simulink model "observer"  (R2014b)
settings: Solver=ode45  StartTime=0.0  StopTime=10.0  RelTol=1e-3
values from neighbouring files (symbols this model uses):
  A11 = A2(1,1)    [zad_8.m]
  A12 = A2(1,2:3)    [zad_8.m]
  A21 = A2(2:3,1)    [zad_8.m]
  A22 = A2(2:3,2:3)    [zad_8.m]
  B_1 = B2(1,1)    [zad_8.m]
  B_2 = B2(2:3,1)    [zad_8.m]
  L = acker(A22',A12', [z2 z3])'    [zad_8.m]
  x0_observer = [ 0 0 ]    [zad_8.m]
undefined symbols (not defined in the file or in its folder): A2, B2, K, Tp, x0
settings Model: Creator=Konrad  LastModifiedBy=Konrad

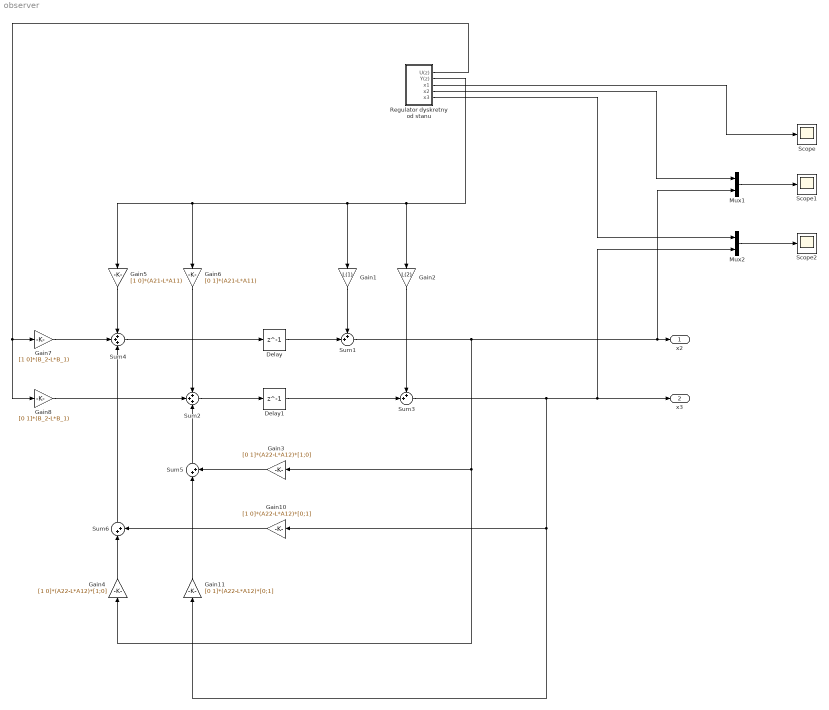
== system observer ==
  Delay : Delay  DelayLength=1  InitialCondition=x0_observer(1)  SampleTime=Tp
  Delay1 : Delay  DelayLength=1  InitialCondition=x0_observer(2)  SampleTime=Tp
  Gain1 : Gain  Gain=L(1)
  Gain10 : Gain  Gain=[1 0]*(A22-L*A12)*[0;1]
  Gain11 : Gain  Gain=[0 1]*(A22-L*A12)*[0;1]
  Gain2 : Gain  Gain=L(2)
  Gain3 : Gain  Gain=[0 1]*(A22-L*A12)*[1;0]
  Gain4 : Gain  Gain=[1 0]*(A22-L*A12)*[1;0]
  Gain5 : Gain  Gain=[1 0]*(A21-L*A11)
  Gain6 : Gain  Gain=[0 1]*(A21-L*A11)
  Gain7 : Gain  Gain=[1 0]*(B_2-L*B_1)
  Gain8 : Gain  Gain=[0 1]*(B_2-L*B_1)
  Mux1 : Mux  Inputs=2
  Mux2 : Mux  Inputs=2
  Regulator dyskretny od stanu : Subsystem
  Scope : Scope
  Scope1 : Scope
  Scope2 : Scope
      settings: SaveName=ScopeData2
  Sum1 : Sum  Inputs=++|
  Sum2 : Sum  Inputs=+++
  Sum3 : Sum  Inputs=++|
  Sum4 : Sum  Inputs=+++
  Sum5 : Sum  Inputs=|++
  Sum6 : Sum  Inputs=|++
  x2 : Outport
  x3 : Outport  Port=2
  wires:
  Delay1/1 -> Sum3/2
  Delay/1 -> Sum1/2
  Regulator dyskretny od stanu/2(Y(z)) -> Gain5/1, Gain6/1, Gain1/1, Gain2/1
  Regulator dyskretny od stanu/1(U(z)) -> Gain8/1, Gain7/1
  Gain3/1 -> Sum5/2
  Gain10/1 -> Sum6/2
  Sum3/1 -> Gain11/1, Gain10/1, Mux2/2, x3/1
  Sum1/1 -> Gain4/1, Gain3/1, Mux1/2, x2/1
  Gain4/1 -> Sum6/1
  Gain11/1 -> Sum5/1
  Gain1/1 -> Sum1/1
  Gain2/1 -> Sum3/1
  Gain5/1 -> Sum4/1
  Gain7/1 -> Sum4/2
  Sum4/1 -> Delay/1
  Sum6/1 -> Sum4/3
  Gain6/1 -> Sum2/1
  Sum2/1 -> Delay1/1
  Sum5/1 -> Sum2/3
  Gain8/1 -> Sum2/2
  Mux1/1 -> Scope1/1
  Mux2/1 -> Scope2/1
  Regulator dyskretny od stanu/4(x2) -> Mux1/1
  Regulator dyskretny od stanu/5(x3) -> Mux2/1
  Regulator dyskretny od stanu/3(x1) -> Scope/1

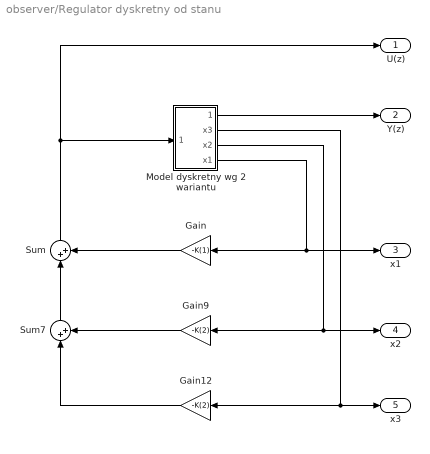
== system observer/Regulator dyskretny od stanu ==
  Gain : Gain  Gain=-K(1)
  Gain12 : Gain  Gain=-K(2)
  Gain9 : Gain  Gain=-K(2)
  Model dyskretny wg 2 wariantu : Subsystem
  Sum : Sum  Inputs=|++
  Sum7 : Sum  Inputs=|++
  U(z) : Outport
  Y(z) : Outport  Port=2
  x1 : Outport  Port=3
  x2 : Outport  Port=4
  x3 : Outport  Port=5
  wires:
  Model dyskretny wg 2 wariantu/1(Y(z)) -> Y(z)/1
  Sum/1 -> U(z)/1, Model dyskretny wg 2 wariantu/1(U(z))
  Gain9/1 -> Sum7/2
  Model dyskretny wg 2 wariantu/4(x1) -> x1/1, Gain/1
  Model dyskretny wg 2 wariantu/2(x3) -> Gain12/1, x3/1
  Sum7/1 -> Sum/1
  Model dyskretny wg 2 wariantu/3(x2) -> Gain9/1, x2/1
  Gain12/1 -> Sum7/1
  Gain/1 -> Sum/2

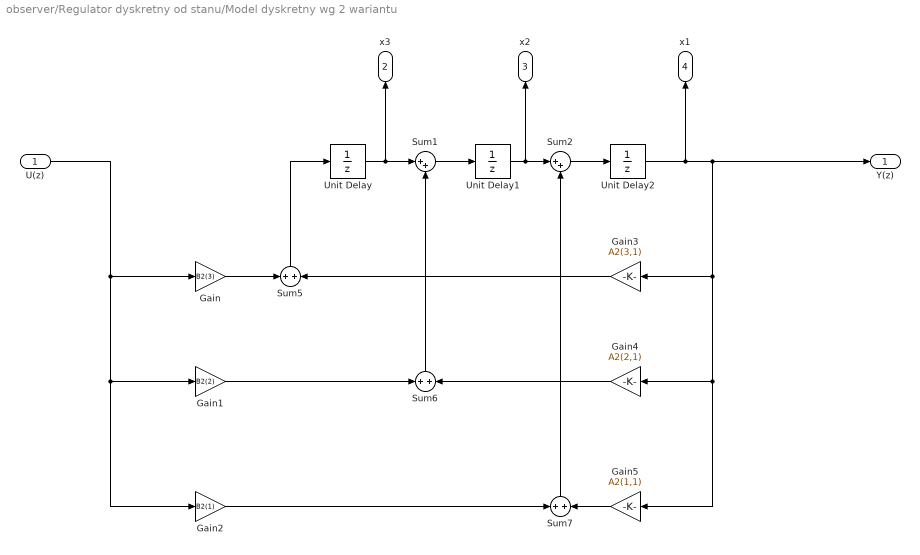
== system observer/Regulator dyskretny od stanu/Model dyskretny wg 2 wariantu ==
  U(z) : Inport
  Gain : Gain  Gain=B2(3)
  Gain1 : Gain  Gain=B2(2)
  Gain2 : Gain  Gain=B2(1)
  Gain3 : Gain  Gain=A2(3,1)
  Gain4 : Gain  Gain=A2(2,1)
  Gain5 : Gain  Gain=A2(1,1)
  Sum1 : Sum  Inputs=|++
  Sum2 : Sum  Inputs=|++
  Sum5 : Sum  Inputs=+|+
  Sum6 : Sum  Inputs=+|+
  Sum7 : Sum  Inputs=+|+
  Unit Delay : UnitDelay  InitialCondition=x0(3)  SampleTime=Tp
  Unit Delay1 : UnitDelay  InitialCondition=x0(2)  SampleTime=Tp
  Unit Delay2 : UnitDelay  InitialCondition=x0(1)  SampleTime=Tp
  Y(z) : Outport
  x3 : Outport  Port=2
  x2 : Outport  Port=3
  x1 : Outport  Port=4
  wires:
  Sum1/1 -> Unit Delay1/1
  Unit Delay1/1 -> x2/1, Sum2/1
  Sum2/1 -> Unit Delay2/1
  Unit Delay/1 -> x3/1, Sum1/1
  Gain1/1 -> Sum6/1
  Gain4/1 -> Sum6/2
  Unit Delay2/1 -> x1/1, Y(z)/1, Gain3/1, Gain4/1, Gain5/1
  Gain3/1 -> Sum5/2
  Gain/1 -> Sum5/1
  Gain5/1 -> Sum7/2
  Sum7/1 -> Sum2/2
  Sum5/1 -> Unit Delay/1
  Gain2/1 -> Sum7/1
  Sum6/1 -> Sum1/2
  U(z)/1 -> Gain/1, Gain1/1, Gain2/1
